simulink model "VCU_CS75_12_30_test"  (R2014a)
settings: Solver=FixedStepDiscrete  StartTime=0.0  StopTime=25  FixedStep=0.0005  RelTol=1e-3
InitFcn:
  | PID_canshu
values from neighbouring files (symbols this model uses):
  D1 = ecucoder_cal(D1)    [PID_canshu.m]
  D2 = ecucoder_cal(D2)    [PID_canshu.m]
  D3 = ecucoder_cal(D3)    [PID_canshu.m]
  ErrorLimit = ecucoder_cal(ErrorLimit)    [PID_canshu.m]
  ErrorSumMax1 = ecucoder_cal(ErrorSumMax1)    [PID_canshu.m]
  ErrorSumMax2 = ecucoder_cal(ErrorSumMax2)    [PID_canshu.m]
  ErrorSumMax3 = ecucoder_cal(ErrorSumMax3)    [PID_canshu.m]
  I1 = ecucoder_cal(I1)    [PID_canshu.m]
  I2 = ecucoder_cal(I2)    [PID_canshu.m]
  I3 = ecucoder_cal(I3)    [PID_canshu.m]
  Limit1 = ecucoder_cal(Limit1)    [PID_canshu.m]
  Limit2 = ecucoder_cal(Limit2)    [PID_canshu.m]
  P1 = ecucoder_cal(P1)    [PID_canshu.m]
  P2 = ecucoder_cal(P2)    [PID_canshu.m]
  P3 = ecucoder_cal(P3)    [PID_canshu.m]
  T_buchang = ecucoder_cal(T_buchang)    [PID_canshu.m]
undefined symbols (not defined in the file or in its folder): ecucoder_acal, I_SW01_L, LaterlAngleCommand, LDW, RemoteAcclPosition
libraries: simulink x940, ec5744lib x41
(part 25 of 31)

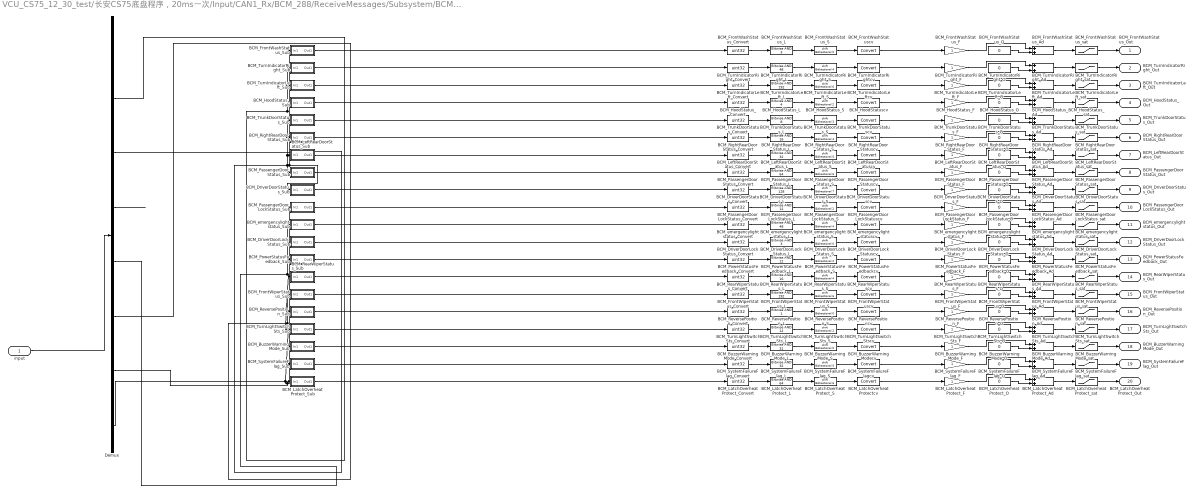
== system VCU_CS75_12_30_test/长安CS75底盘程序，20ms一次/Input/CAN1_Rx/BCM_288/ReceiveMessages/Subsystem/BCM_1 ==
  input : Inport
  BCM_BuzzerWarningMode_Ad : Sum
  BCM_BuzzerWarningMode_Convert : DataTypeConversion  OutDataTypeStr=uint32
  BCM_BuzzerWarningMode_F : Gain
  BCM_BuzzerWarningMode_L : simulink/Logic and Bit Operations/Bitwise Operator  logicop=AND  UseBitMask=on  BitMask=31  BitMaskRealWorld=Stored Integer
  BCM_BuzzerWarningMode_O : Constant  Value=0  OutDataTypeStr=single
  BCM_BuzzerWarningMode_S : ArithShift
  BCM_BuzzerWarningMode_Sub : Subsystem
  BCM_BuzzerWarningMode_sat : Saturate  UpperLimit=31  LowerLimit=0
  BCM_BuzzerWarningModecv : DataTypeConversion
  BCM_DriverDoorLockStatus_Ad : Sum
  BCM_DriverDoorLockStatus_Convert : DataTypeConversion  OutDataTypeStr=uint32
  BCM_DriverDoorLockStatus_F : Gain
  BCM_DriverDoorLockStatus_L : simulink/Logic and Bit Operations/Bitwise Operator  logicop=AND  UseBitMask=on  BitMask=3  BitMaskRealWorld=Stored Integer
  BCM_DriverDoorLockStatus_O : Constant  Value=0  OutDataTypeStr=single
  BCM_DriverDoorLockStatus_S : ArithShift
  BCM_DriverDoorLockStatus_Sub : Subsystem
  BCM_DriverDoorLockStatus_sat : Saturate  UpperLimit=3  LowerLimit=0
  BCM_DriverDoorLockStatuscv : DataTypeConversion
  BCM_DriverDoorStatus_Ad : Sum
  BCM_DriverDoorStatus_Convert : DataTypeConversion  OutDataTypeStr=uint32
  BCM_DriverDoorStatus_F : Gain
  BCM_DriverDoorStatus_L : simulink/Logic and Bit Operations/Bitwise Operator  logicop=AND  UseBitMask=on  BitMask=128  BitMaskRealWorld=Stored Integer
  BCM_DriverDoorStatus_O : Constant  Value=0  OutDataTypeStr=single
  BCM_DriverDoorStatus_S : ArithShift  BitShiftNumber=7
  BCM_DriverDoorStatus_Sub : Subsystem
  BCM_DriverDoorStatus_sat : Saturate  UpperLimit=1  LowerLimit=0
  BCM_DriverDoorStatuscv : DataTypeConversion
  BCM_FrontWashStatus_Ad : Sum
  BCM_FrontWashStatus_Convert : DataTypeConversion  OutDataTypeStr=uint32
  BCM_FrontWashStatus_F : Gain
  BCM_FrontWashStatus_L : simulink/Logic and Bit Operations/Bitwise Operator  logicop=AND  UseBitMask=on  BitMask=3  BitMaskRealWorld=Stored Integer
  BCM_FrontWashStatus_O : Constant  Value=0  OutDataTypeStr=single
  BCM_FrontWashStatus_S : ArithShift
  BCM_FrontWashStatus_Sub : Subsystem
  BCM_FrontWashStatus_sat : Saturate  UpperLimit=3  LowerLimit=0
  BCM_FrontWashStatuscv : DataTypeConversion
  BCM_FrontWiperStatus_Ad : Sum
  BCM_FrontWiperStatus_Convert : DataTypeConversion  OutDataTypeStr=uint32
  BCM_FrontWiperStatus_F : Gain
  BCM_FrontWiperStatus_L : simulink/Logic and Bit Operations/Bitwise Operator  logicop=AND  UseBitMask=on  BitMask=192  BitMaskRealWorld=Stored Integer
  BCM_FrontWiperStatus_O : Constant  Value=0  OutDataTypeStr=single
  BCM_FrontWiperStatus_S : ArithShift  BitShiftNumber=6
  BCM_FrontWiperStatus_Sub : Subsystem
  BCM_FrontWiperStatus_sat : Saturate  UpperLimit=3  LowerLimit=0
  BCM_FrontWiperStatuscv : DataTypeConversion
  BCM_HoodStatus_Ad : Sum
  BCM_HoodStatus_Convert : DataTypeConversion  OutDataTypeStr=uint32
  BCM_HoodStatus_F : Gain
  BCM_HoodStatus_L : simulink/Logic and Bit Operations/Bitwise Operator  logicop=AND  UseBitMask=on  BitMask=4  BitMaskRealWorld=Stored Integer
  BCM_HoodStatus_O : Constant  Value=0  OutDataTypeStr=single
  BCM_HoodStatus_S : ArithShift  BitShiftNumber=2
  BCM_HoodStatus_Sub : Subsystem
  BCM_HoodStatus_sat : Saturate  UpperLimit=1  LowerLimit=0
  BCM_HoodStatuscv : DataTypeConversion
  BCM_LatchOverheatProtect_Ad : Sum
  BCM_LatchOverheatProtect_Convert : DataTypeConversion  OutDataTypeStr=uint32
  BCM_LatchOverheatProtect_F : Gain
  BCM_LatchOverheatProtect_L : simulink/Logic and Bit Operations/Bitwise Operator  logicop=AND  UseBitMask=on  BitMask=64  BitMaskRealWorld=Stored Integer
  BCM_LatchOverheatProtect_O : Constant  Value=0  OutDataTypeStr=single
  BCM_LatchOverheatProtect_S : ArithShift  BitShiftNumber=6
  BCM_LatchOverheatProtect_Sub : Subsystem
  BCM_LatchOverheatProtect_sat : Saturate  UpperLimit=1  LowerLimit=0
  BCM_LatchOverheatProtectcv : DataTypeConversion
  BCM_LeftRearDoorStatus_Ad : Sum
  BCM_LeftRearDoorStatus_Convert : DataTypeConversion  OutDataTypeStr=uint32
  BCM_LeftRearDoorStatus_F : Gain
  BCM_LeftRearDoorStatus_L : simulink/Logic and Bit Operations/Bitwise Operator  logicop=AND  UseBitMask=on  BitMask=32  BitMaskRealWorld=Stored Integer
  BCM_LeftRearDoorStatus_O : Constant  Value=0  OutDataTypeStr=single
  BCM_LeftRearDoorStatus_S : ArithShift  BitShiftNumber=5
  BCM_LeftRearDoorStatus_Sub : Subsystem
  BCM_LeftRearDoorStatus_sat : Saturate  UpperLimit=1  LowerLimit=0
  BCM_LeftRearDoorStatuscv : DataTypeConversion
  BCM_PassengerDoorLockStatus_Ad : Sum
  BCM_PassengerDoorLockStatus_Convert : DataTypeConversion  OutDataTypeStr=uint32
  BCM_PassengerDoorLockStatus_F : Gain
  BCM_PassengerDoorLockStatus_L : simulink/Logic and Bit Operations/Bitwise Operator  logicop=AND  UseBitMask=on  BitMask=12  BitMaskRealWorld=Stored Integer
  BCM_PassengerDoorLockStatus_O : Constant  Value=0  OutDataTypeStr=single
  BCM_PassengerDoorLockStatus_S : ArithShift  BitShiftNumber=2
  BCM_PassengerDoorLockStatus_Sub : Subsystem
  BCM_PassengerDoorLockStatus_sat : Saturate  UpperLimit=3  LowerLimit=0
  BCM_PassengerDoorLockStatuscv : DataTypeConversion
  BCM_PassengerDoorStatus_Ad : Sum
  BCM_PassengerDoorStatus_Convert : DataTypeConversion  OutDataTypeStr=uint32
  BCM_PassengerDoorStatus_F : Gain
  BCM_PassengerDoorStatus_L : simulink/Logic and Bit Operations/Bitwise Operator  logicop=AND  UseBitMask=on  BitMask=64  BitMaskRealWorld=Stored Integer
  BCM_PassengerDoorStatus_O : Constant  Value=0  OutDataTypeStr=single
  BCM_PassengerDoorStatus_S : ArithShift  BitShiftNumber=6
  BCM_PassengerDoorStatus_Sub : Subsystem
  BCM_PassengerDoorStatus_sat : Saturate  UpperLimit=1  LowerLimit=0
  BCM_PassengerDoorStatuscv : DataTypeConversion
  BCM_PowerStatusFeedback_Ad : Sum
  BCM_PowerStatusFeedback_Convert : DataTypeConversion  OutDataTypeStr=uint32
  BCM_PowerStatusFeedback_F : Gain
  BCM_PowerStatusFeedback_L : simulink/Logic and Bit Operations/Bitwise Operator  logicop=AND  UseBitMask=on  BitMask=12  BitMaskRealWorld=Stored Integer
  BCM_PowerStatusFeedback_O : Constant  Value=0  OutDataTypeStr=single
  BCM_PowerStatusFeedback_S : ArithShift  BitShiftNumber=2
  BCM_PowerStatusFeedback_Sub : Subsystem
  BCM_PowerStatusFeedback_sat : Saturate  UpperLimit=3  LowerLimit=0
  BCM_PowerStatusFeedbackcv : DataTypeConversion
  BCM_RearWiperStatus_Ad : Sum
  BCM_RearWiperStatus_Convert : DataTypeConversion  OutDataTypeStr=uint32
  BCM_RearWiperStatus_F : Gain
  BCM_RearWiperStatus_L : simulink/Logic and Bit Operations/Bitwise Operator  logicop=AND  UseBitMask=on  BitMask=16  BitMaskRealWorld=Stored Integer
  BCM_RearWiperStatus_O : Constant  Value=0  OutDataTypeStr=single
  BCM_RearWiperStatus_S : ArithShift  BitShiftNumber=4
  BCM_RearWiperStatus_Sub : Subsystem
  BCM_RearWiperStatus_sat : Saturate  UpperLimit=1  LowerLimit=0
  BCM_RearWiperStatuscv : DataTypeConversion
  BCM_ReversePosition_Ad : Sum
  BCM_ReversePosition_Convert : DataTypeConversion  OutDataTypeStr=uint32
  BCM_ReversePosition_F : Gain
  BCM_ReversePosition_L : simulink/Logic and Bit Operations/Bitwise Operator  logicop=AND  UseBitMask=on  BitMask=1  BitMaskRealWorld=Stored Integer
  BCM_ReversePosition_O : Constant  Value=0  OutDataTypeStr=single
  BCM_ReversePosition_S : ArithShift
  BCM_ReversePosition_Sub : Subsystem
  BCM_ReversePosition_sat : Saturate  UpperLimit=1  LowerLimit=0
  BCM_ReversePositioncv : DataTypeConversion
  BCM_RightRearDoorStatus_Ad : Sum
  BCM_RightRearDoorStatus_Convert : DataTypeConversion  OutDataTypeStr=uint32
  BCM_RightRearDoorStatus_F : Gain
  BCM_RightRearDoorStatus_L : simulink/Logic and Bit Operations/Bitwise Operator  logicop=AND  UseBitMask=on  BitMask=16  BitMaskRealWorld=Stored Integer
  BCM_RightRearDoorStatus_O : Constant  Value=0  OutDataTypeStr=single
  BCM_RightRearDoorStatus_S : ArithShift  BitShiftNumber=4
  BCM_RightRearDoorStatus_Sub : Subsystem
  BCM_RightRearDoorStatus_sat : Saturate  UpperLimit=1  LowerLimit=0
  BCM_RightRearDoorStatuscv : DataTypeConversion
  BCM_SystemFailureFlag_Ad : Sum
  BCM_SystemFailureFlag_Convert : DataTypeConversion  OutDataTypeStr=uint32
  BCM_SystemFailureFlag_F : Gain
  BCM_SystemFailureFlag_L : simulink/Logic and Bit Operations/Bitwise Operator  logicop=AND  UseBitMask=on  BitMask=32  BitMaskRealWorld=Stored Integer
  BCM_SystemFailureFlag_O : Constant  Value=0  OutDataTypeStr=single
  BCM_SystemFailureFlag_S : ArithShift  BitShiftNumber=5
  BCM_SystemFailureFlag_Sub : Subsystem
  BCM_SystemFailureFlag_sat : Saturate  UpperLimit=1  LowerLimit=0
  BCM_SystemFailureFlagcv : DataTypeConversion
  BCM_TrunkDoorStatus_Ad : Sum
  BCM_TrunkDoorStatus_Convert : DataTypeConversion  OutDataTypeStr=uint32
  BCM_TrunkDoorStatus_F : Gain
  BCM_TrunkDoorStatus_L : simulink/Logic and Bit Operations/Bitwise Operator  logicop=AND  UseBitMask=on  BitMask=8  BitMaskRealWorld=Stored Integer
  BCM_TrunkDoorStatus_O : Constant  Value=0  OutDataTypeStr=single
  BCM_TrunkDoorStatus_S : ArithShift  BitShiftNumber=3
  BCM_TrunkDoorStatus_Sub : Subsystem
  BCM_TrunkDoorStatus_sat : Saturate  UpperLimit=1  LowerLimit=0
  BCM_TrunkDoorStatuscv : DataTypeConversion
  BCM_TurnIndicatorLeft_Ad : Sum
  BCM_TurnIndicatorLeft_Convert : DataTypeConversion  OutDataTypeStr=uint32
  BCM_TurnIndicatorLeft_F : Gain
  BCM_TurnIndicatorLeft_L : simulink/Logic and Bit Operations/Bitwise Operator  logicop=AND  UseBitMask=on  BitMask=192  BitMaskRealWorld=Stored Integer
  BCM_TurnIndicatorLeft_O : Constant  Value=0  OutDataTypeStr=single
  BCM_TurnIndicatorLeft_S : ArithShift  BitShiftNumber=6
  BCM_TurnIndicatorLeft_Sub : Subsystem
  BCM_TurnIndicatorLeft_sat : Saturate  UpperLimit=3  LowerLimit=0
  BCM_TurnIndicatorLeftcv : DataTypeConversion
  BCM_TurnIndicatorRight_Ad : Sum
  BCM_TurnIndicatorRight_Convert : DataTypeConversion  OutDataTypeStr=uint32
  BCM_TurnIndicatorRight_F : Gain
  BCM_TurnIndicatorRight_L : simulink/Logic and Bit Operations/Bitwise Operator  logicop=AND  UseBitMask=on  BitMask=48  BitMaskRealWorld=Stored Integer
  BCM_TurnIndicatorRight_O : Constant  Value=0  OutDataTypeStr=single
  BCM_TurnIndicatorRight_S : ArithShift  BitShiftNumber=4
  BCM_TurnIndicatorRight_Sub : Subsystem
  BCM_TurnIndicatorRight_sat : Saturate  UpperLimit=3  LowerLimit=0
  BCM_TurnIndicatorRightcv : DataTypeConversion
  BCM_TurnLightSwitchSts_Ad : Sum
  BCM_TurnLightSwitchSts_Convert : DataTypeConversion  OutDataTypeStr=uint32
  BCM_TurnLightSwitchSts_F : Gain
  BCM_TurnLightSwitchSts_L : simulink/Logic and Bit Operations/Bitwise Operator  logicop=AND  UseBitMask=on  BitMask=12  BitMaskRealWorld=Stored Integer
  BCM_TurnLightSwitchSts_O : Constant  Value=0  OutDataTypeStr=single
  BCM_TurnLightSwitchSts_S : ArithShift  BitShiftNumber=2
  BCM_TurnLightSwitchSts_Sub : Subsystem
  BCM_TurnLightSwitchSts_sat : Saturate  UpperLimit=3  LowerLimit=0
  BCM_TurnLightSwitchStscv : DataTypeConversion
  BCM_emergencylightstatus_Ad : Sum
  BCM_emergencylightstatus_Convert : DataTypeConversion  OutDataTypeStr=uint32
  BCM_emergencylightstatus_F : Gain
  BCM_emergencylightstatus_L : simulink/Logic and Bit Operations/Bitwise Operator  logicop=AND  UseBitMask=on  BitMask=48  BitMaskRealWorld=Stored Integer
  BCM_emergencylightstatus_O : Constant  Value=0  OutDataTypeStr=single
  BCM_emergencylightstatus_S : ArithShift  BitShiftNumber=4
  BCM_emergencylightstatus_Sub : Subsystem
  BCM_emergencylightstatus_sat : Saturate  UpperLimit=3  LowerLimit=0
  BCM_emergencylightstatuscv : DataTypeConversion
  Demux : Demux  Outputs=8
  BCM_FrontWashStatus_Out : Outport
  BCM_TurnIndicatorRight_Out : Outport  Port=2
  BCM_TurnIndicatorLeft_Out : Outport  Port=3
  BCM_HoodStatus_Out : Outport  Port=4
  BCM_TrunkDoorStatus_Out : Outport  Port=5
  BCM_RightRearDoorStatus_Out : Outport  Port=6
  BCM_LeftRearDoorStatus_Out : Outport  Port=7
  BCM_PassengerDoorStatus_Out : Outport  Port=8
  BCM_DriverDoorStatus_Out : Outport  Port=9
  BCM_PassengerDoorLockStatus_Out : Outport  Port=10
  BCM_emergencylightstatus_Out : Outport  Port=11
  BCM_DriverDoorLockStatus_Out : Outport  Port=12
  BCM_PowerStatusFeedback_Out : Outport  Port=13
  BCM_RearWiperStatus_Out : Outport  Port=14
  BCM_FrontWiperStatus_Out : Outport  Port=15
  BCM_ReversePosition_Out : Outport  Port=16
  BCM_TurnLightSwitchSts_Out : Outport  Port=17
  BCM_BuzzerWarningMode_Out : Outport  Port=18
  BCM_SystemFailureFlag_Out : Outport  Port=19
  BCM_LatchOverheatProtect_Out : Outport  Port=20
  wires:
  input/1 -> Demux/1
  BCM_LatchOverheatProtectcv/1 -> BCM_LatchOverheatProtect_F/1
  BCM_LatchOverheatProtect_S/1 -> BCM_LatchOverheatProtectcv/1
  BCM_LatchOverheatProtect_L/1 -> BCM_LatchOverheatProtect_S/1
  BCM_LatchOverheatProtect_Convert/1 -> BCM_LatchOverheatProtect_L/1
  BCM_LatchOverheatProtect_Sub/1(Out1) -> BCM_LatchOverheatProtect_Convert/1
  BCM_LatchOverheatProtect_sat/1 -> BCM_LatchOverheatProtect_Out/1
  BCM_LatchOverheatProtect_Ad/1 -> BCM_LatchOverheatProtect_sat/1
  BCM_LatchOverheatProtect_O/1 -> BCM_LatchOverheatProtect_Ad/2
  BCM_LatchOverheatProtect_F/1 -> BCM_LatchOverheatProtect_Ad/1
  BCM_SystemFailureFlagcv/1 -> BCM_SystemFailureFlag_F/1
  BCM_SystemFailureFlag_S/1 -> BCM_SystemFailureFlagcv/1
  BCM_SystemFailureFlag_L/1 -> BCM_SystemFailureFlag_S/1
  BCM_SystemFailureFlag_Convert/1 -> BCM_SystemFailureFlag_L/1
  BCM_SystemFailureFlag_Sub/1(Out1) -> BCM_SystemFailureFlag_Convert/1
  BCM_SystemFailureFlag_sat/1 -> BCM_SystemFailureFlag_Out/1
  BCM_SystemFailureFlag_Ad/1 -> BCM_SystemFailureFlag_sat/1
  BCM_SystemFailureFlag_O/1 -> BCM_SystemFailureFlag_Ad/2
  BCM_SystemFailureFlag_F/1 -> BCM_SystemFailureFlag_Ad/1
  BCM_BuzzerWarningModecv/1 -> BCM_BuzzerWarningMode_F/1
  BCM_BuzzerWarningMode_S/1 -> BCM_BuzzerWarningModecv/1
  BCM_BuzzerWarningMode_L/1 -> BCM_BuzzerWarningMode_S/1
  BCM_BuzzerWarningMode_Convert/1 -> BCM_BuzzerWarningMode_L/1
  BCM_BuzzerWarningMode_Sub/1(Out1) -> BCM_BuzzerWarningMode_Convert/1
  Demux/8 -> BCM_SystemFailureFlag_Sub/1(In1), BCM_BuzzerWarningMode_Sub/1(In1), BCM_LatchOverheatProtect_Sub/1(In1)
  BCM_BuzzerWarningMode_sat/1 -> BCM_BuzzerWarningMode_Out/1
  BCM_BuzzerWarningMode_Ad/1 -> BCM_BuzzerWarningMode_sat/1
  BCM_BuzzerWarningMode_O/1 -> BCM_BuzzerWarningMode_Ad/2
  BCM_BuzzerWarningMode_F/1 -> BCM_BuzzerWarningMode_Ad/1
  BCM_TurnLightSwitchStscv/1 -> BCM_TurnLightSwitchSts_F/1
  BCM_TurnLightSwitchSts_S/1 -> BCM_TurnLightSwitchStscv/1
  BCM_TurnLightSwitchSts_L/1 -> BCM_TurnLightSwitchSts_S/1
  BCM_TurnLightSwitchSts_Convert/1 -> BCM_TurnLightSwitchSts_L/1
  BCM_TurnLightSwitchSts_Sub/1(Out1) -> BCM_TurnLightSwitchSts_Convert/1
  BCM_TurnLightSwitchSts_sat/1 -> BCM_TurnLightSwitchSts_Out/1
  BCM_TurnLightSwitchSts_Ad/1 -> BCM_TurnLightSwitchSts_sat/1
  BCM_TurnLightSwitchSts_O/1 -> BCM_TurnLightSwitchSts_Ad/2
  BCM_TurnLightSwitchSts_F/1 -> BCM_TurnLightSwitchSts_Ad/1
  BCM_ReversePositioncv/1 -> BCM_ReversePosition_F/1
  BCM_ReversePosition_S/1 -> BCM_ReversePositioncv/1
  BCM_ReversePosition_L/1 -> BCM_ReversePosition_S/1
  BCM_ReversePosition_Convert/1 -> BCM_ReversePosition_L/1
  BCM_ReversePosition_Sub/1(Out1) -> BCM_ReversePosition_Convert/1
  Demux/7 -> BCM_TurnLightSwitchSts_Sub/1(In1), BCM_ReversePosition_Sub/1(In1)
  BCM_ReversePosition_sat/1 -> BCM_ReversePosition_Out/1
  BCM_ReversePosition_Ad/1 -> BCM_ReversePosition_sat/1
  BCM_ReversePosition_O/1 -> BCM_ReversePosition_Ad/2
  BCM_ReversePosition_F/1 -> BCM_ReversePosition_Ad/1
  BCM_FrontWiperStatuscv/1 -> BCM_FrontWiperStatus_F/1
  BCM_FrontWiperStatus_S/1 -> BCM_FrontWiperStatuscv/1
  BCM_FrontWiperStatus_L/1 -> BCM_FrontWiperStatus_S/1
  BCM_FrontWiperStatus_Convert/1 -> BCM_FrontWiperStatus_L/1
  BCM_FrontWiperStatus_Sub/1(Out1) -> BCM_FrontWiperStatus_Convert/1
  BCM_FrontWiperStatus_sat/1 -> BCM_FrontWiperStatus_Out/1
  BCM_FrontWiperStatus_Ad/1 -> BCM_FrontWiperStatus_sat/1
  BCM_FrontWiperStatus_O/1 -> BCM_FrontWiperStatus_Ad/2
  BCM_FrontWiperStatus_F/1 -> BCM_FrontWiperStatus_Ad/1
  BCM_RearWiperStatuscv/1 -> BCM_RearWiperStatus_F/1
  BCM_RearWiperStatus_S/1 -> BCM_RearWiperStatuscv/1
  BCM_RearWiperStatus_L/1 -> BCM_RearWiperStatus_S/1
  BCM_RearWiperStatus_Convert/1 -> BCM_RearWiperStatus_L/1
  BCM_RearWiperStatus_Sub/1(Out1) -> BCM_RearWiperStatus_Convert/1
  BCM_RearWiperStatus_sat/1 -> BCM_RearWiperStatus_Out/1
  BCM_RearWiperStatus_Ad/1 -> BCM_RearWiperStatus_sat/1
  BCM_RearWiperStatus_O/1 -> BCM_RearWiperStatus_Ad/2
  BCM_RearWiperStatus_F/1 -> BCM_RearWiperStatus_Ad/1
  BCM_PowerStatusFeedbackcv/1 -> BCM_PowerStatusFeedback_F/1
  BCM_PowerStatusFeedback_S/1 -> BCM_PowerStatusFeedbackcv/1
  BCM_PowerStatusFeedback_L/1 -> BCM_PowerStatusFeedback_S/1
  BCM_PowerStatusFeedback_Convert/1 -> BCM_PowerStatusFeedback_L/1
  BCM_PowerStatusFeedback_Sub/1(Out1) -> BCM_PowerStatusFeedback_Convert/1
  BCM_PowerStatusFeedback_sat/1 -> BCM_PowerStatusFeedback_Out/1
  BCM_PowerStatusFeedback_Ad/1 -> BCM_PowerStatusFeedback_sat/1
  BCM_PowerStatusFeedback_O/1 -> BCM_PowerStatusFeedback_Ad/2
  BCM_PowerStatusFeedback_F/1 -> BCM_PowerStatusFeedback_Ad/1
  BCM_DriverDoorLockStatuscv/1 -> BCM_DriverDoorLockStatus_F/1
  BCM_DriverDoorLockStatus_S/1 -> BCM_DriverDoorLockStatuscv/1
  BCM_DriverDoorLockStatus_L/1 -> BCM_DriverDoorLockStatus_S/1
  BCM_DriverDoorLockStatus_Convert/1 -> BCM_DriverDoorLockStatus_L/1
  BCM_DriverDoorLockStatus_Sub/1(Out1) -> BCM_DriverDoorLockStatus_Convert/1
  Demux/6 -> BCM_PowerStatusFeedback_Sub/1(In1), BCM_DriverDoorLockStatus_Sub/1(In1), BCM_RearWiperStatus_Sub/1(In1), BCM_FrontWiperStatus_Sub/1(In1)
  BCM_DriverDoorLockStatus_sat/1 -> BCM_DriverDoorLockStatus_Out/1
  BCM_DriverDoorLockStatus_Ad/1 -> BCM_DriverDoorLockStatus_sat/1
  BCM_DriverDoorLockStatus_O/1 -> BCM_DriverDoorLockStatus_Ad/2
  BCM_DriverDoorLockStatus_F/1 -> BCM_DriverDoorLockStatus_Ad/1
  BCM_emergencylightstatuscv/1 -> BCM_emergencylightstatus_F/1
  BCM_emergencylightstatus_S/1 -> BCM_emergencylightstatuscv/1
  BCM_emergencylightstatus_L/1 -> BCM_emergencylightstatus_S/1
  BCM_emergencylightstatus_Convert/1 -> BCM_emergencylightstatus_L/1
  BCM_emergencylightstatus_Sub/1(Out1) -> BCM_emergencylightstatus_Convert/1
  BCM_emergencylightstatus_sat/1 -> BCM_emergencylightstatus_Out/1
  BCM_emergencylightstatus_Ad/1 -> BCM_emergencylightstatus_sat/1
  BCM_emergencylightstatus_O/1 -> BCM_emergencylightstatus_Ad/2
  BCM_emergencylightstatus_F/1 -> BCM_emergencylightstatus_Ad/1
  BCM_PassengerDoorLockStatuscv/1 -> BCM_PassengerDoorLockStatus_F/1
  BCM_PassengerDoorLockStatus_S/1 -> BCM_PassengerDoorLockStatuscv/1
  BCM_PassengerDoorLockStatus_L/1 -> BCM_PassengerDoorLockStatus_S/1
  BCM_PassengerDoorLockStatus_Convert/1 -> BCM_PassengerDoorLockStatus_L/1
  BCM_PassengerDoorLockStatus_Sub/1(Out1) -> BCM_PassengerDoorLockStatus_Convert/1
  Demux/5 -> BCM_emergencylightstatus_Sub/1(In1), BCM_PassengerDoorLockStatus_Sub/1(In1)
  BCM_PassengerDoorLockStatus_sat/1 -> BCM_PassengerDoorLockStatus_Out/1
  BCM_PassengerDoorLockStatus_Ad/1 -> BCM_PassengerDoorLockStatus_sat/1
  BCM_PassengerDoorLockStatus_O/1 -> BCM_PassengerDoorLockStatus_Ad/2
  BCM_PassengerDoorLockStatus_F/1 -> BCM_PassengerDoorLockStatus_Ad/1
  BCM_DriverDoorStatuscv/1 -> BCM_DriverDoorStatus_F/1
  BCM_DriverDoorStatus_S/1 -> BCM_DriverDoorStatuscv/1
  BCM_DriverDoorStatus_L/1 -> BCM_DriverDoorStatus_S/1
  BCM_DriverDoorStatus_Convert/1 -> BCM_DriverDoorStatus_L/1
  BCM_DriverDoorStatus_Sub/1(Out1) -> BCM_DriverDoorStatus_Convert/1
  BCM_DriverDoorStatus_sat/1 -> BCM_DriverDoorStatus_Out/1
  BCM_DriverDoorStatus_Ad/1 -> BCM_DriverDoorStatus_sat/1
  BCM_DriverDoorStatus_O/1 -> BCM_DriverDoorStatus_Ad/2
  BCM_DriverDoorStatus_F/1 -> BCM_DriverDoorStatus_Ad/1
  BCM_PassengerDoorStatuscv/1 -> BCM_PassengerDoorStatus_F/1
  BCM_PassengerDoorStatus_S/1 -> BCM_PassengerDoorStatuscv/1
  BCM_PassengerDoorStatus_L/1 -> BCM_PassengerDoorStatus_S/1
  BCM_PassengerDoorStatus_Convert/1 -> BCM_PassengerDoorStatus_L/1
  BCM_PassengerDoorStatus_Sub/1(Out1) -> BCM_PassengerDoorStatus_Convert/1
  BCM_PassengerDoorStatus_sat/1 -> BCM_PassengerDoorStatus_Out/1
  BCM_PassengerDoorStatus_Ad/1 -> BCM_PassengerDoorStatus_sat/1
  BCM_PassengerDoorStatus_O/1 -> BCM_PassengerDoorStatus_Ad/2
  BCM_PassengerDoorStatus_F/1 -> BCM_PassengerDoorStatus_Ad/1
  BCM_LeftRearDoorStatuscv/1 -> BCM_LeftRearDoorStatus_F/1
  BCM_LeftRearDoorStatus_S/1 -> BCM_LeftRearDoorStatuscv/1
  BCM_LeftRearDoorStatus_L/1 -> BCM_LeftRearDoorStatus_S/1
  BCM_LeftRearDoorStatus_Convert/1 -> BCM_LeftRearDoorStatus_L/1
  BCM_LeftRearDoorStatus_Sub/1(Out1) -> BCM_LeftRearDoorStatus_Convert/1
  BCM_LeftRearDoorStatus_sat/1 -> BCM_LeftRearDoorStatus_Out/1
  BCM_LeftRearDoorStatus_Ad/1 -> BCM_LeftRearDoorStatus_sat/1
  BCM_LeftRearDoorStatus_O/1 -> BCM_LeftRearDoorStatus_Ad/2
  BCM_LeftRearDoorStatus_F/1 -> BCM_LeftRearDoorStatus_Ad/1
  BCM_RightRearDoorStatuscv/1 -> BCM_RightRearDoorStatus_F/1
  BCM_RightRearDoorStatus_S/1 -> BCM_RightRearDoorStatuscv/1
  BCM_RightRearDoorStatus_L/1 -> BCM_RightRearDoorStatus_S/1
  BCM_RightRearDoorStatus_Convert/1 -> BCM_RightRearDoorStatus_L/1
  BCM_RightRearDoorStatus_Sub/1(Out1) -> BCM_RightRearDoorStatus_Convert/1
  BCM_RightRearDoorStatus_sat/1 -> BCM_RightRearDoorStatus_Out/1
  BCM_RightRearDoorStatus_Ad/1 -> BCM_RightRearDoorStatus_sat/1
  BCM_RightRearDoorStatus_O/1 -> BCM_RightRearDoorStatus_Ad/2
  BCM_RightRearDoorStatus_F/1 -> BCM_RightRearDoorStatus_Ad/1
  BCM_TrunkDoorStatuscv/1 -> BCM_TrunkDoorStatus_F/1
  BCM_TrunkDoorStatus_S/1 -> BCM_TrunkDoorStatuscv/1
  BCM_TrunkDoorStatus_L/1 -> BCM_TrunkDoorStatus_S/1
  BCM_TrunkDoorStatus_Convert/1 -> BCM_TrunkDoorStatus_L/1
  BCM_TrunkDoorStatus_Sub/1(Out1) -> BCM_TrunkDoorStatus_Convert/1
  BCM_TrunkDoorStatus_sat/1 -> BCM_TrunkDoorStatus_Out/1
  BCM_TrunkDoorStatus_Ad/1 -> BCM_TrunkDoorStatus_sat/1
  BCM_TrunkDoorStatus_O/1 -> BCM_TrunkDoorStatus_Ad/2
  BCM_TrunkDoorStatus_F/1 -> BCM_TrunkDoorStatus_Ad/1
  BCM_HoodStatuscv/1 -> BCM_HoodStatus_F/1
  BCM_HoodStatus_S/1 -> BCM_HoodStatuscv/1
  BCM_HoodStatus_L/1 -> BCM_HoodStatus_S/1
  BCM_HoodStatus_Convert/1 -> BCM_HoodStatus_L/1
  BCM_HoodStatus_Sub/1(Out1) -> BCM_HoodStatus_Convert/1
  Demux/3 -> BCM_DriverDoorStatus_Sub/1(In1), BCM_HoodStatus_Sub/1(In1), BCM_RightRearDoorStatus_Sub/1(In1), BCM_TrunkDoorStatus_Sub/1(In1), BCM_LeftRearDoorStatus_Sub/1(In1), BCM_PassengerDoorStatus_Sub/1(In1)
  BCM_HoodStatus_sat/1 -> BCM_HoodStatus_Out/1
  BCM_HoodStatus_Ad/1 -> BCM_HoodStatus_sat/1
  BCM_HoodStatus_O/1 -> BCM_HoodStatus_Ad/2
  BCM_HoodStatus_F/1 -> BCM_HoodStatus_Ad/1
  BCM_TurnIndicatorLeftcv/1 -> BCM_TurnIndicatorLeft_F/1
  BCM_TurnIndicatorLeft_S/1 -> BCM_TurnIndicatorLeftcv/1
  BCM_TurnIndicatorLeft_L/1 -> BCM_TurnIndicatorLeft_S/1
  BCM_TurnIndicatorLeft_Convert/1 -> BCM_TurnIndicatorLeft_L/1
  BCM_TurnIndicatorLeft_Sub/1(Out1) -> BCM_TurnIndicatorLeft_Convert/1
  BCM_TurnIndicatorLeft_sat/1 -> BCM_TurnIndicatorLeft_Out/1
  BCM_TurnIndicatorLeft_Ad/1 -> BCM_TurnIndicatorLeft_sat/1
  BCM_TurnIndicatorLeft_O/1 -> BCM_TurnIndicatorLeft_Ad/2
  BCM_TurnIndicatorLeft_F/1 -> BCM_TurnIndicatorLeft_Ad/1
  BCM_TurnIndicatorRightcv/1 -> BCM_TurnIndicatorRight_F/1
  BCM_TurnIndicatorRight_S/1 -> BCM_TurnIndicatorRightcv/1
  BCM_TurnIndicatorRight_L/1 -> BCM_TurnIndicatorRight_S/1
  BCM_TurnIndicatorRight_Convert/1 -> BCM_TurnIndicatorRight_L/1
  BCM_TurnIndicatorRight_Sub/1(Out1) -> BCM_TurnIndicatorRight_Convert/1
  BCM_TurnIndicatorRight_sat/1 -> BCM_TurnIndicatorRight_Out/1
  BCM_TurnIndicatorRight_Ad/1 -> BCM_TurnIndicatorRight_sat/1
  BCM_TurnIndicatorRight_O/1 -> BCM_TurnIndicatorRight_Ad/2
  BCM_TurnIndicatorRight_F/1 -> BCM_TurnIndicatorRight_Ad/1
  BCM_FrontWashStatuscv/1 -> BCM_FrontWashStatus_F/1
  BCM_FrontWashStatus_S/1 -> BCM_FrontWashStatuscv/1
  BCM_FrontWashStatus_L/1 -> BCM_FrontWashStatus_S/1
  BCM_FrontWashStatus_Convert/1 -> BCM_FrontWashStatus_L/1
  BCM_FrontWashStatus_Sub/1(Out1) -> BCM_FrontWashStatus_Convert/1
  Demux/2 -> BCM_TurnIndicatorLeft_Sub/1(In1), BCM_TurnIndicatorRight_Sub/1(In1), BCM_FrontWashStatus_Sub/1(In1)
  BCM_FrontWashStatus_sat/1 -> BCM_FrontWashStatus_Out/1
  BCM_FrontWashStatus_Ad/1 -> BCM_FrontWashStatus_sat/1
  BCM_FrontWashStatus_O/1 -> BCM_FrontWashStatus_Ad/2
  BCM_FrontWashStatus_F/1 -> BCM_FrontWashStatus_Ad/1
  Demux/4 -> ?

== system VCU_CS75_12_30_test/长安CS75底盘程序，20ms一次/Input/CAN1_Rx/BCM_328/ReceiveMessages/Subsystem/BCM_1 ==
  input : Inport
  Demux : Demux  Outputs=8
  LCM_DRLSts_Ad : Sum
  LCM_DRLSts_Convert : DataTypeConversion  OutDataTypeStr=uint32
  LCM_DRLSts_F : Gain
  LCM_DRLSts_L : simulink/Logic and Bit Operations/Bitwise Operator  logicop=AND  UseBitMask=on  BitMask=192  BitMaskRealWorld=Stored Integer
  LCM_DRLSts_O : Constant  Value=0  OutDataTypeStr=single
  LCM_DRLSts_S : ArithShift  BitShiftNumber=6
  LCM_DRLSts_Sub : Subsystem
  LCM_DRLSts_sat : Saturate  UpperLimit=0  LowerLimit=0
  LCM_DRLStscv : DataTypeConversion
  LCM_DriveMode_Ad : Sum
  LCM_DriveMode_Convert : DataTypeConversion  OutDataTypeStr=uint32
  LCM_DriveMode_F : Gain
  LCM_DriveMode_L : simulink/Logic and Bit Operations/Bitwise Operator  logicop=AND  UseBitMask=on  BitMask=192  BitMaskRealWorld=Stored Integer
  LCM_DriveMode_O : Constant  Value=0  OutDataTypeStr=single
  LCM_DriveMode_S : ArithShift  BitShiftNumber=6
  LCM_DriveMode_Sub : Subsystem
  LCM_DriveMode_sat : Saturate  UpperLimit=0  LowerLimit=0
  LCM_DriveModecv : DataTypeConversion
  LCM_LASSwitch_Ad : Sum
  LCM_LASSwitch_Convert : DataTypeConversion  OutDataTypeStr=uint32
  LCM_LASSwitch_F : Gain
  LCM_LASSwitch_L : simulink/Logic and Bit Operations/Bitwise Operator  logicop=AND  UseBitMask=on  BitMask=3  BitMaskRealWorld=Stored Integer
  LCM_LASSwitch_O : Constant  Value=0  OutDataTypeStr=single
  LCM_LASSwitch_S : ArithShift
  LCM_LASSwitch_Sub : Subsystem
  LCM_LASSwitch_sat : Saturate  UpperLimit=3  LowerLimit=0
  LCM_LASSwitchcv : DataTypeConversion
  LCM_RearLeftTuningLightFaultSts_Ad : Sum
  LCM_RearLeftTuningLightFaultSts_Convert : DataTypeConversion  OutDataTypeStr=uint32
  LCM_RearLeftTuningLightFaultSts_F : Gain
  LCM_RearLeftTuningLightFaultSts_L : simulink/Logic and Bit Operations/Bitwise Operator  logicop=AND  UseBitMask=on  BitMask=128  BitMaskRealWorld=Stored Integer
  LCM_RearLeftTuningLightFaultSts_O : Constant  Value=0  OutDataTypeStr=single
  LCM_RearLeftTuningLightFaultSts_S : ArithShift  BitShiftNumber=7
  LCM_RearLeftTuningLightFaultSts_Sub : Subsystem
  LCM_RearLeftTuningLightFaultSts_sat : Saturate  UpperLimit=0  LowerLimit=0
  LCM_RearLeftTuningLightFaultStscv : DataTypeConversion
  LCM_RearRightTuningLightFaultSts_Ad : Sum
  LCM_RearRightTuningLightFaultSts_Convert : DataTypeConversion  OutDataTypeStr=uint32
  LCM_RearRightTuningLightFaultSts_F : Gain
  LCM_RearRightTuningLightFaultSts_L : simulink/Logic and Bit Operations/Bitwise Operator  logicop=AND  UseBitMask=on  BitMask=128  BitMaskRealWorld=Stored Integer
  LCM_RearRightTuningLightFaultSts_O : Constant  Value=0  OutDataTypeStr=single
  LCM_RearRightTuningLightFaultSts_S : ArithShift  BitShiftNumber=7
  LCM_RearRightTuningLightFaultSts_Sub : Subsystem
  LCM_RearRightTuningLightFaultSts_sat : Saturate  UpperLimit=0  LowerLimit=0
  LCM_RearRightTuningLightFaultStscv : DataTypeConversion
  LCM_ReverseLightSts_Ad : Sum
  LCM_ReverseLightSts_Convert : DataTypeConversion  OutDataTypeStr=uint32
  LCM_ReverseLightSts_F : Gain
  LCM_ReverseLightSts_L : simulink/Logic and Bit Operations/Bitwise Operator  logicop=AND  UseBitMask=on  BitMask=192  BitMaskRealWorld=Stored Integer
  LCM_ReverseLightSts_O : Constant  Value=0  OutDataTypeStr=single
  LCM_ReverseLightSts_S : ArithShift  BitShiftNumber=6
  LCM_ReverseLightSts_Sub : Subsystem
  LCM_ReverseLightSts_sat : Saturate  UpperLimit=0  LowerLimit=0
  LCM_ReverseLightStscv : DataTypeConversion
  LCM_DriveMode_Out : Outport
  LCM_DRLSts_Out : Outport  Port=2
  LCM_LASSwitch_Out : Outport  Port=3
  LCM_RearRightTuningLightFaultSts_Out : Outport  Port=4
  LCM_RearLeftTuningLightFaultSts_Out : Outport  Port=5
  LCM_ReverseLightSts_Out : Outport  Port=6
  wires:
  input/1 -> Demux/1
  LCM_ReverseLightStscv/1 -> LCM_ReverseLightSts_F/1
  LCM_ReverseLightSts_S/1 -> LCM_ReverseLightStscv/1
  LCM_ReverseLightSts_L/1 -> LCM_ReverseLightSts_S/1
  LCM_ReverseLightSts_Convert/1 -> LCM_ReverseLightSts_L/1
  LCM_ReverseLightSts_Sub/1(Out1) -> LCM_ReverseLightSts_Convert/1
  Demux/6 -> LCM_ReverseLightSts_Sub/1(In1)
  LCM_ReverseLightSts_sat/1 -> LCM_ReverseLightSts_Out/1
  LCM_ReverseLightSts_Ad/1 -> LCM_ReverseLightSts_sat/1
  LCM_ReverseLightSts_O/1 -> LCM_ReverseLightSts_Ad/2
  LCM_ReverseLightSts_F/1 -> LCM_ReverseLightSts_Ad/1
  LCM_RearLeftTuningLightFaultStscv/1 -> LCM_RearLeftTuningLightFaultSts_F/1
  LCM_RearLeftTuningLightFaultSts_S/1 -> LCM_RearLeftTuningLightFaultStscv/1
  LCM_RearLeftTuningLightFaultSts_L/1 -> LCM_RearLeftTuningLightFaultSts_S/1
  LCM_RearLeftTuningLightFaultSts_Convert/1 -> LCM_RearLeftTuningLightFaultSts_L/1
  LCM_RearLeftTuningLightFaultSts_Sub/1(Out1) -> LCM_RearLeftTuningLightFaultSts_Convert/1
  Demux/5 -> LCM_RearLeftTuningLightFaultSts_Sub/1(In1)
  LCM_RearLeftTuningLightFaultSts_sat/1 -> LCM_RearLeftTuningLightFaultSts_Out/1
  LCM_RearLeftTuningLightFaultSts_Ad/1 -> LCM_RearLeftTuningLightFaultSts_sat/1
  LCM_RearLeftTuningLightFaultSts_O/1 -> LCM_RearLeftTuningLightFaultSts_Ad/2
  LCM_RearLeftTuningLightFaultSts_F/1 -> LCM_RearLeftTuningLightFaultSts_Ad/1
  LCM_RearRightTuningLightFaultStscv/1 -> LCM_RearRightTuningLightFaultSts_F/1
  LCM_RearRightTuningLightFaultSts_S/1 -> LCM_RearRightTuningLightFaultStscv/1
  LCM_RearRightTuningLightFaultSts_L/1 -> LCM_RearRightTuningLightFaultSts_S/1
  LCM_RearRightTuningLightFaultSts_Convert/1 -> LCM_RearRightTuningLightFaultSts_L/1
  LCM_RearRightTuningLightFaultSts_Sub/1(Out1) -> LCM_RearRightTuningLightFaultSts_Convert/1
  Demux/4 -> LCM_RearRightTuningLightFaultSts_Sub/1(In1)
  LCM_RearRightTuningLightFaultSts_sat/1 -> LCM_RearRightTuningLightFaultSts_Out/1
  LCM_RearRightTuningLightFaultSts_Ad/1 -> LCM_RearRightTuningLightFaultSts_sat/1
  LCM_RearRightTuningLightFaultSts_O/1 -> LCM_RearRightTuningLightFaultSts_Ad/2
  LCM_RearRightTuningLightFaultSts_F/1 -> LCM_RearRightTuningLightFaultSts_Ad/1
  LCM_LASSwitchcv/1 -> LCM_LASSwitch_F/1
  LCM_LASSwitch_S/1 -> LCM_LASSwitchcv/1
  LCM_LASSwitch_L/1 -> LCM_LASSwitch_S/1
  LCM_LASSwitch_Convert/1 -> LCM_LASSwitch_L/1
  LCM_LASSwitch_Sub/1(Out1) -> LCM_LASSwitch_Convert/1
  Demux/3 -> LCM_LASSwitch_Sub/1(In1)
  LCM_LASSwitch_sat/1 -> LCM_LASSwitch_Out/1
  LCM_LASSwitch_Ad/1 -> LCM_LASSwitch_sat/1
  LCM_LASSwitch_O/1 -> LCM_LASSwitch_Ad/2
  LCM_LASSwitch_F/1 -> LCM_LASSwitch_Ad/1
  LCM_DRLStscv/1 -> LCM_DRLSts_F/1
  LCM_DRLSts_S/1 -> LCM_DRLStscv/1
  LCM_DRLSts_L/1 -> LCM_DRLSts_S/1
  LCM_DRLSts_Convert/1 -> LCM_DRLSts_L/1
  LCM_DRLSts_Sub/1(Out1) -> LCM_DRLSts_Convert/1
  Demux/2 -> LCM_DRLSts_Sub/1(In1)
  LCM_DRLSts_sat/1 -> LCM_DRLSts_Out/1
  LCM_DRLSts_Ad/1 -> LCM_DRLSts_sat/1
  LCM_DRLSts_O/1 -> LCM_DRLSts_Ad/2
  LCM_DRLSts_F/1 -> LCM_DRLSts_Ad/1
  LCM_DriveModecv/1 -> LCM_DriveMode_F/1
  LCM_DriveMode_S/1 -> LCM_DriveModecv/1
  LCM_DriveMode_L/1 -> LCM_DriveMode_S/1
  LCM_DriveMode_Convert/1 -> LCM_DriveMode_L/1
  LCM_DriveMode_Sub/1(Out1) -> LCM_DriveMode_Convert/1
  Demux/1 -> LCM_DriveMode_Sub/1(In1)
  LCM_DriveMode_sat/1 -> LCM_DriveMode_Out/1
  LCM_DriveMode_Ad/1 -> LCM_DriveMode_sat/1
  LCM_DriveMode_O/1 -> LCM_DriveMode_Ad/2
  LCM_DriveMode_F/1 -> LCM_DriveMode_Ad/1

== system VCU_CS75_12_30_test/长安CS75底盘程序，20ms一次/Input/CAN1_Rx/BCM_348/ReceiveMessages/Subsystem/BCM_1 ==
  input : Inport
  BCM_DriveMode_Ad : Sum
  BCM_DriveMode_Convert : DataTypeConversion  OutDataTypeStr=uint32
  BCM_DriveMode_F : Gain
  BCM_DriveMode_L : simulink/Logic and Bit Operations/Bitwise Operator  logicop=AND  UseBitMask=on  BitMask=6  BitMaskRealWorld=Stored Integer
  BCM_DriveMode_O : Constant  Value=0  OutDataTypeStr=single
  BCM_DriveMode_S : ArithShift  BitShiftNumber=1
  BCM_DriveMode_Sub : Subsystem
  BCM_DriveMode_sat : Saturate  UpperLimit=3  LowerLimit=0
  BCM_DriveModecv : DataTypeConversion
  BCM_LockSignal_Ad : Sum
  BCM_LockSignal_Convert : DataTypeConversion  OutDataTypeStr=uint32
  BCM_LockSignal_F : Gain
  BCM_LockSignal_L : simulink/Logic and Bit Operations/Bitwise Operator  logicop=AND  UseBitMask=on  BitMask=24  BitMaskRealWorld=Stored Integer
  BCM_LockSignal_O : Constant  Value=0  OutDataTypeStr=single
  BCM_LockSignal_S : ArithShift  BitShiftNumber=3
  BCM_LockSignal_Sub : Subsystem
  BCM_LockSignal_sat : Saturate  UpperLimit=3  LowerLimit=0
  BCM_LockSignalcv : DataTypeConversion
  BCM_UnlockSignal_Ad : Sum
  BCM_UnlockSignal_Convert : DataTypeConversion  OutDataTypeStr=uint32
  BCM_UnlockSignal_F : Gain
  BCM_UnlockSignal_L : simulink/Logic and Bit Operations/Bitwise Operator  logicop=AND  UseBitMask=on  BitMask=96  BitMaskRealWorld=Stored Integer
  BCM_UnlockSignal_O : Constant  Value=0  OutDataTypeStr=single
  BCM_UnlockSignal_S : ArithShift  BitShiftNumber=5
  BCM_UnlockSignal_Sub : Subsystem
  BCM_UnlockSignal_sat : Saturate  UpperLimit=3  LowerLimit=0
  BCM_UnlockSignalcv : DataTypeConversion
  Demux : Demux  Outputs=8
  BCM_DriveMode_Out : Outport
  BCM_LockSignal_Out : Outport  Port=2
  BCM_UnlockSignal_Out : Outport  Port=3
  wires:
  input/1 -> Demux/1
  BCM_UnlockSignalcv/1 -> BCM_UnlockSignal_F/1
  BCM_UnlockSignal_S/1 -> BCM_UnlockSignalcv/1
  BCM_UnlockSignal_L/1 -> BCM_UnlockSignal_S/1
  BCM_UnlockSignal_Convert/1 -> BCM_UnlockSignal_L/1
  BCM_UnlockSignal_Sub/1(Out1) -> BCM_UnlockSignal_Convert/1
  BCM_UnlockSignal_sat/1 -> BCM_UnlockSignal_Out/1
  BCM_UnlockSignal_Ad/1 -> BCM_UnlockSignal_sat/1
  BCM_UnlockSignal_O/1 -> BCM_UnlockSignal_Ad/2
  BCM_UnlockSignal_F/1 -> BCM_UnlockSignal_Ad/1
  BCM_LockSignalcv/1 -> BCM_LockSignal_F/1
  BCM_LockSignal_S/1 -> BCM_LockSignalcv/1
  BCM_LockSignal_L/1 -> BCM_LockSignal_S/1
  BCM_LockSignal_Convert/1 -> BCM_LockSignal_L/1
  BCM_LockSignal_Sub/1(Out1) -> BCM_LockSignal_Convert/1
  BCM_LockSignal_sat/1 -> BCM_LockSignal_Out/1
  BCM_LockSignal_Ad/1 -> BCM_LockSignal_sat/1
  BCM_LockSignal_O/1 -> BCM_LockSignal_Ad/2
  BCM_LockSignal_F/1 -> BCM_LockSignal_Ad/1
  BCM_DriveModecv/1 -> BCM_DriveMode_F/1
  BCM_DriveMode_S/1 -> BCM_DriveModecv/1
  BCM_DriveMode_L/1 -> BCM_DriveMode_S/1
  BCM_DriveMode_Convert/1 -> BCM_DriveMode_L/1
  BCM_DriveMode_Sub/1(Out1) -> BCM_DriveMode_Convert/1
  Demux/6 -> BCM_UnlockSignal_Sub/1(In1), BCM_LockSignal_Sub/1(In1), BCM_DriveMode_Sub/1(In1)
  BCM_DriveMode_sat/1 -> BCM_DriveMode_Out/1
  BCM_DriveMode_Ad/1 -> BCM_DriveMode_sat/1
  BCM_DriveMode_O/1 -> BCM_DriveMode_Ad/2
  BCM_DriveMode_F/1 -> BCM_DriveMode_Ad/1

== system VCU_CS75_12_30_test/长安CS75底盘程序，20ms一次/Input/CAN1_Rx/BCM_3DF/ReceiveMessages/Subsystem/BCM_3DF1 ==
  input : Inport
  BCM_AmbientLightColorFeedback_Ad : Sum
  BCM_AmbientLightColorFeedback_Convert : DataTypeConversion  OutDataTypeStr=uint32
  BCM_AmbientLightColorFeedback_F : Gain
  BCM_AmbientLightColorFeedback_L : simulink/Logic and Bit Operations/Bitwise Operator  logicop=AND  UseBitMask=on  BitMask=255  BitMaskRealWorld=Stored Integer
  BCM_AmbientLightColorFeedback_O : Constant  Value=0  OutDataTypeStr=single
  BCM_AmbientLightColorFeedback_S : ArithShift
  BCM_AmbientLightColorFeedback_Sub : Subsystem
  BCM_AmbientLightColorFeedback_sat : Saturate  UpperLimit=255  LowerLimit=0
  BCM_AmbientLightColorFeedbackcv : DataTypeConversion
  BCM_CRC_Checksum_Ad : Sum
  BCM_CRC_Checksum_Convert : DataTypeConversion  OutDataTypeStr=uint32
  BCM_CRC_Checksum_F : Gain
  BCM_CRC_Checksum_L : simulink/Logic and Bit Operations/Bitwise Operator  logicop=AND  UseBitMask=on  BitMask=255  BitMaskRealWorld=Stored Integer
  BCM_CRC_Checksum_O : Constant  Value=0  OutDataTypeStr=single
  BCM_CRC_Checksum_S : ArithShift
  BCM_CRC_Checksum_Sub : Subsystem
  BCM_CRC_Checksum_sat : Saturate  UpperLimit=0  LowerLimit=0
  BCM_CRC_Checksumcv : DataTypeConversion
  BCM_DriveModeFeedback_Ad : Sum
  BCM_DriveModeFeedback_Convert : DataTypeConversion  OutDataTypeStr=uint32
  BCM_DriveModeFeedback_F : Gain
  BCM_DriveModeFeedback_L : simulink/Logic and Bit Operations/Bitwise Operator  logicop=AND  UseBitMask=on  BitMask=48  BitMaskRealWorld=Stored Integer
  BCM_DriveModeFeedback_O : Constant  Value=0  OutDataTypeStr=single
  BCM_DriveModeFeedback_S : ArithShift  BitShiftNumber=4
  BCM_DriveModeFeedback_Sub : Subsystem
  BCM_DriveModeFeedback_sat : Saturate  UpperLimit=3  LowerLimit=0
  BCM_DriveModeFeedbackcv : DataTypeConversion
  BCM_DriveModeStatus_Ad : Sum
  BCM_DriveModeStatus_Convert : DataTypeConversion  OutDataTypeStr=uint32
  BCM_DriveModeStatus_F : Gain
  BCM_DriveModeStatus_L : simulink/Logic and Bit Operations/Bitwise Operator  logicop=AND  UseBitMask=on  BitMask=15  BitMaskRealWorld=Stored Integer
  BCM_DriveModeStatus_O : Constant  Value=0  OutDataTypeStr=single
  BCM_DriveModeStatus_S : ArithShift
  BCM_DriveModeStatus_Sub : Subsystem
  BCM_DriveModeStatus_sat : Saturate  UpperLimit=15  LowerLimit=0
  BCM_DriveModeStatuscv : DataTypeConversion
  BCM_DriveMode_Ad : Sum
  BCM_DriveMode_Convert : DataTypeConversion  OutDataTypeStr=uint32
  BCM_DriveMode_F : Gain
  BCM_DriveMode_L : simulink/Logic and Bit Operations/Bitwise Operator  logicop=AND  UseBitMask=on  BitMask=240  BitMaskRealWorld=Stored Integer
  BCM_DriveMode_O : Constant  Value=0  OutDataTypeStr=single
  BCM_DriveMode_S : ArithShift  BitShiftNumber=4
  BCM_DriveMode_Sub : Subsystem
  BCM_DriveMode_sat : Saturate  UpperLimit=0  LowerLimit=0
  BCM_DriveModecv : DataTypeConversion
  BCM_EPSTorqueModeFeedback_Ad : Sum
  BCM_EPSTorqueModeFeedback_Convert : DataTypeConversion  OutDataTypeStr=uint32
  BCM_EPSTorqueModeFeedback_F : Gain
  BCM_EPSTorqueModeFeedback_L : simulink/Logic and Bit Operations/Bitwise Operator  logicop=AND  UseBitMask=on  BitMask=192  BitMaskRealWorld=Stored Integer
  BCM_EPSTorqueModeFeedback_O : Constant  Value=0  OutDataTypeStr=single
  BCM_EPSTorqueModeFeedback_S : ArithShift  BitShiftNumber=6
  BCM_EPSTorqueModeFeedback_Sub : Subsystem
  BCM_EPSTorqueModeFeedback_sat : Saturate  UpperLimit=3  LowerLimit=0
  BCM_EPSTorqueModeFeedbackcv : DataTypeConversion
  BCM_EPSTorqueMode_Ad : Sum
  BCM_EPSTorqueMode_Convert : DataTypeConversion  OutDataTypeStr=uint32
  BCM_EPSTorqueMode_F : Gain
  BCM_EPSTorqueMode_L : simulink/Logic and Bit Operations/Bitwise Operator  logicop=AND  UseBitMask=on  BitMask=6  BitMaskRealWorld=Stored Integer
  BCM_EPSTorqueMode_O : Constant  Value=0  OutDataTypeStr=single
  BCM_EPSTorqueMode_S : ArithShift  BitShiftNumber=1
  BCM_EPSTorqueMode_Sub : Subsystem
  BCM_EPSTorqueMode_sat : Saturate  UpperLimit=3  LowerLimit=0
  BCM_EPSTorqueModecv : DataTypeConversion
  BCM_RollingCounter_Ad : Sum
  BCM_RollingCounter_Convert : DataTypeConversion  OutDataTypeStr=uint32
  BCM_RollingCounter_F : Gain
  BCM_RollingCounter_L : simulink/Logic and Bit Operations/Bitwise Operator  logicop=AND  UseBitMask=on  BitMask=15  BitMaskRealWorld=Stored Integer
  BCM_RollingCounter_O : Constant  Value=0  OutDataTypeStr=single
  BCM_RollingCounter_S : ArithShift
  BCM_RollingCounter_Sub : Subsystem
  BCM_RollingCounter_sat : Saturate  UpperLimit=0  LowerLimit=0
  BCM_RollingCountercv : DataTypeConversion
  Demux : Demux  Outputs=8
  BCM_DriveMode_Out : Outport
  BCM_EPSTorqueMode_Out : Outport  Port=2
  BCM_DriveModeStatus_Out : Outport  Port=3
  BCM_DriveModeFeedback_Out : Outport  Port=4
  BCM_EPSTorqueModeFeedback_Out : Outport  Port=5
  BCM_AmbientLightColorFeedback_Out : Outport  Port=6
  BCM_RollingCounter_Out : Outport  Port=7
  BCM_CRC_Checksum_Out : Outport  Port=8
  wires:
  input/1 -> Demux/1
  BCM_CRC_Checksumcv/1 -> BCM_CRC_Checksum_F/1
  BCM_CRC_Checksum_S/1 -> BCM_CRC_Checksumcv/1
  BCM_CRC_Checksum_L/1 -> BCM_CRC_Checksum_S/1
  BCM_CRC_Checksum_Convert/1 -> BCM_CRC_Checksum_L/1
  BCM_CRC_Checksum_Sub/1(Out1) -> BCM_CRC_Checksum_Convert/1
  Demux/8 -> BCM_CRC_Checksum_Sub/1(In1)
  BCM_CRC_Checksum_sat/1 -> BCM_CRC_Checksum_Out/1
  BCM_CRC_Checksum_Ad/1 -> BCM_CRC_Checksum_sat/1
  BCM_CRC_Checksum_O/1 -> BCM_CRC_Checksum_Ad/2
  BCM_CRC_Checksum_F/1 -> BCM_CRC_Checksum_Ad/1
  BCM_RollingCountercv/1 -> BCM_RollingCounter_F/1
  BCM_RollingCounter_S/1 -> BCM_RollingCountercv/1
  BCM_RollingCounter_L/1 -> BCM_RollingCounter_S/1
  BCM_RollingCounter_Convert/1 -> BCM_RollingCounter_L/1
  BCM_RollingCounter_Sub/1(Out1) -> BCM_RollingCounter_Convert/1
  Demux/7 -> BCM_RollingCounter_Sub/1(In1)
  BCM_RollingCounter_sat/1 -> BCM_RollingCounter_Out/1
  BCM_RollingCounter_Ad/1 -> BCM_RollingCounter_sat/1
  BCM_RollingCounter_O/1 -> BCM_RollingCounter_Ad/2
  BCM_RollingCounter_F/1 -> BCM_RollingCounter_Ad/1
  BCM_AmbientLightColorFeedbackcv/1 -> BCM_AmbientLightColorFeedback_F/1
  BCM_AmbientLightColorFeedback_S/1 -> BCM_AmbientLightColorFeedbackcv/1
  BCM_AmbientLightColorFeedback_L/1 -> BCM_AmbientLightColorFeedback_S/1
  BCM_AmbientLightColorFeedback_Convert/1 -> BCM_AmbientLightColorFeedback_L/1
  BCM_AmbientLightColorFeedback_Sub/1(Out1) -> BCM_AmbientLightColorFeedback_Convert/1
  Demux/4 -> BCM_AmbientLightColorFeedback_Sub/1(In1)
  BCM_AmbientLightColorFeedback_sat/1 -> BCM_AmbientLightColorFeedback_Out/1
  BCM_AmbientLightColorFeedback_Ad/1 -> BCM_AmbientLightColorFeedback_sat/1
  BCM_AmbientLightColorFeedback_O/1 -> BCM_AmbientLightColorFeedback_Ad/2
  BCM_AmbientLightColorFeedback_F/1 -> BCM_AmbientLightColorFeedback_Ad/1
  BCM_EPSTorqueModeFeedbackcv/1 -> BCM_EPSTorqueModeFeedback_F/1
  BCM_EPSTorqueModeFeedback_S/1 -> BCM_EPSTorqueModeFeedbackcv/1
  BCM_EPSTorqueModeFeedback_L/1 -> BCM_EPSTorqueModeFeedback_S/1
  BCM_EPSTorqueModeFeedback_Convert/1 -> BCM_EPSTorqueModeFeedback_L/1
  BCM_EPSTorqueModeFeedback_Sub/1(Out1) -> BCM_EPSTorqueModeFeedback_Convert/1
  BCM_EPSTorqueModeFeedback_sat/1 -> BCM_EPSTorqueModeFeedback_Out/1
  BCM_EPSTorqueModeFeedback_Ad/1 -> BCM_EPSTorqueModeFeedback_sat/1
  BCM_EPSTorqueModeFeedback_O/1 -> BCM_EPSTorqueModeFeedback_Ad/2
  BCM_EPSTorqueModeFeedback_F/1 -> BCM_EPSTorqueModeFeedback_Ad/1
  BCM_DriveModeFeedbackcv/1 -> BCM_DriveModeFeedback_F/1
  BCM_DriveModeFeedback_S/1 -> BCM_DriveModeFeedbackcv/1
  BCM_DriveModeFeedback_L/1 -> BCM_DriveModeFeedback_S/1
  BCM_DriveModeFeedback_Convert/1 -> BCM_DriveModeFeedback_L/1
  BCM_DriveModeFeedback_Sub/1(Out1) -> BCM_DriveModeFeedback_Convert/1
  BCM_DriveModeFeedback_sat/1 -> BCM_DriveModeFeedback_Out/1
  BCM_DriveModeFeedback_Ad/1 -> BCM_DriveModeFeedback_sat/1
  BCM_DriveModeFeedback_O/1 -> BCM_DriveModeFeedback_Ad/2
  BCM_DriveModeFeedback_F/1 -> BCM_DriveModeFeedback_Ad/1
  BCM_DriveModeStatuscv/1 -> BCM_DriveModeStatus_F/1
  BCM_DriveModeStatus_S/1 -> BCM_DriveModeStatuscv/1
  BCM_DriveModeStatus_L/1 -> BCM_DriveModeStatus_S/1
  BCM_DriveModeStatus_Convert/1 -> BCM_DriveModeStatus_L/1
  BCM_DriveModeStatus_Sub/1(Out1) -> BCM_DriveModeStatus_Convert/1
  Demux/3 -> BCM_EPSTorqueModeFeedback_Sub/1(In1), BCM_DriveModeFeedback_Sub/1(In1), BCM_DriveModeStatus_Sub/1(In1)
  BCM_DriveModeStatus_sat/1 -> BCM_DriveModeStatus_Out/1
  BCM_DriveModeStatus_Ad/1 -> BCM_DriveModeStatus_sat/1
  BCM_DriveModeStatus_O/1 -> BCM_DriveModeStatus_Ad/2
  BCM_DriveModeStatus_F/1 -> BCM_DriveModeStatus_Ad/1
  BCM_EPSTorqueModecv/1 -> BCM_EPSTorqueMode_F/1
  BCM_EPSTorqueMode_S/1 -> BCM_EPSTorqueModecv/1
  BCM_EPSTorqueMode_L/1 -> BCM_EPSTorqueMode_S/1
  BCM_EPSTorqueMode_Convert/1 -> BCM_EPSTorqueMode_L/1
  BCM_EPSTorqueMode_Sub/1(Out1) -> BCM_EPSTorqueMode_Convert/1
  Demux/2 -> BCM_EPSTorqueMode_Sub/1(In1)
  BCM_EPSTorqueMode_sat/1 -> BCM_EPSTorqueMode_Out/1
  BCM_EPSTorqueMode_Ad/1 -> BCM_EPSTorqueMode_sat/1
  BCM_EPSTorqueMode_O/1 -> BCM_EPSTorqueMode_Ad/2
  BCM_EPSTorqueMode_F/1 -> BCM_EPSTorqueMode_Ad/1
  BCM_DriveModecv/1 -> BCM_DriveMode_F/1
  BCM_DriveMode_S/1 -> BCM_DriveModecv/1
  BCM_DriveMode_L/1 -> BCM_DriveMode_S/1
  BCM_DriveMode_Convert/1 -> BCM_DriveMode_L/1
  BCM_DriveMode_Sub/1(Out1) -> BCM_DriveMode_Convert/1
  Demux/1 -> BCM_DriveMode_Sub/1(In1)
  BCM_DriveMode_sat/1 -> BCM_DriveMode_Out/1
  BCM_DriveMode_Ad/1 -> BCM_DriveMode_sat/1
  BCM_DriveMode_O/1 -> BCM_DriveMode_Ad/2
  BCM_DriveMode_F/1 -> BCM_DriveMode_Ad/1
